simulink model "jessilll"  (R2021a)
settings: Solver=VariableStepAuto  StartTime=0.0  StopTime=500  RelTol=1e-3
settings Model: Creator=USER  LastModifiedBy=User

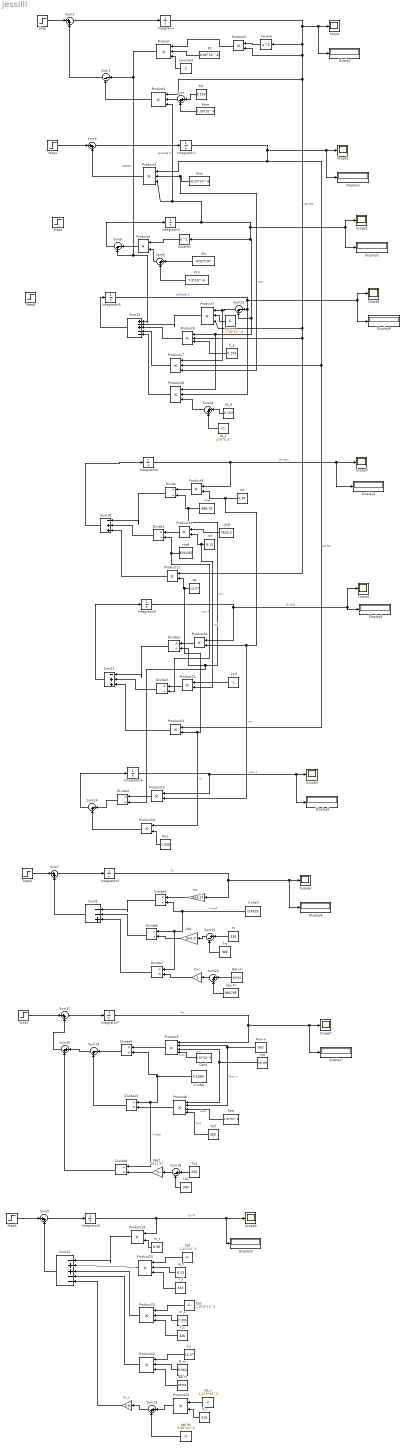
== system jessilll ==
  Constant : Constant  Value=2
  Cp_v : Constant  Value=2.373*10^3
  Cpc : Constant  Value=1.814*10^3
  Cpf : Constant  Value=1.22*10^3
  Cpv Tr : Constant  Value=984795
  Cpw : Constant  Value=1.87*10^3
  Cpw1 : Constant  Value=1.87*10^3
  Del Hv : Constant  Value=69781
  Display{,1..9} (10 alike) : Display
  Divide{,1..5,9} (7 alike) : Product  Inputs=*/
  Divide{6..8,10} (4 alike) : Product  Inputs=/*
  Integrator{,1..2,6..9} (7 alike) : Integrator
  Integrator3 : Integrator  InitialCondition=415
  Integrator4 : Integrator  InitialCondition=7632.2
  Integrator5 : Integrator  InitialCondition=587.47
  K_p : Constant  Value=0.193
  Kp : Constant  Value=0.193
  Kt_c : Constant  Value=47075.07
  Kt_d : Constant  Value=0.193
  Ktc : Constant  Value=47075.07
  Ktd : Constant  Value=7.3*10^-6
  Kti : Constant  Value=8.86*10^-20
  Ktrm : Constant  Value=7.39*10^-6
  Ktrm_1 : Constant  Value=7.39*10^-6
  Ktrs : Constant  Value=-8.25*10^-6
  Product{,1,3,7..8,17..18,20..22} (10 alike) : Product  Inputs=3
  Product{2,4,9..16,19,23} (12 alike) : Product
  Product5 : Product  Inputs=4
  Product6 : Product  Inputs=4
  R_m : Constant  Value=8.964
  Row w : Constant  Value=997
  Ru1 : Constant  Value=1.008
  Scope{,1..9} (10 alike) : Scope
  Square : Math  Operator=square  SaturateOnIntegerOverflow=on
  Square1 : Math  Operator=square  SaturateOnIntegerOverflow=on
  Step : Step  Time=0  Before=0.001  After=0.25  SampleTime=0
  Step1 : Step  Time=0  Before=0.001  After=0.01  SampleTime=0
  Step{2..4,8} (4 alike) : Step  SampleTime=0
  Step7 : Step  After=326  SampleTime=0
  Sum{,2..3,5,7,9,13,16..17,20,24} (11 alike) : Sum  Inputs=|++
  Sum1 : Sum  Inputs=|--
  Sum10 : Sum  Inputs=|-++
  Sum11 : Sum  Inputs=|-++
  Sum12 : Sum  Inputs=|-++--
  Sum{6,14,19,22} (4 alike) : Sum  Inputs=|-+
  Sum15 : Sum  Inputs=|+-
  Sum18 : Sum  Inputs=|+-
  Sum23 : Sum  Inputs=|+-+--
  Sum8 : Sum  Inputs=|--+
  T_c : Constant  Value=326
  T_f : Constant  Value=333
  T_r : Constant  Value=415
  Tc : Constant  Value=326
  Tc1 : Constant  Value=326
  Tw : Constant  Value=300
  Tw1 : Constant  Value=300
  Twf : Constant  Value=300
  UAc : Gain  Gain=3842.37
  UAc1 : Gain  Gain=3842.37
  V shell : Constant  Value=0.4919
  V tube : Constant  Value=0.1094
  VR : Constant  Value=14.07
  V_r : Constant  Value=14.07
  "[M]f" : Constant  Value=7632.2
  "[S]f" : Constant
  del H : Constant  Value=69781
  del Hv : Constant  Value=6.99*10^4
  m_c : Constant  Value=0.305
  m_f : Constant  Value=6.13
  m_t : Constant  Value=6.39
  m_v : Gain  Gain=3.96
  mc : Gain  Gain=553.27
  mf : Constant  Value=6.13
  mt : Constant  Value=6.39
  mv : Gain
  mw : Constant  Value=59.09
  row : Constant  Value=986.76
  rowf : Constant  Value=858.085
  wires:
  Integrator/1 -> Display/1, Scope/1, Product7/3, Product8/2, Product11/1, Product1/1, Product2/2, Square/1  "[M] RM"
  Kti/1 -> Product/2
  Constant/1 -> Product/3
  Kp/1 -> Sum/1
  Ktrm/1 -> Sum/2
  Sum/1 -> Product1/2
  Product/1 -> Sum6/2, Sum23/1, Sum1/1  "2Kti[M]"
  Product1/1 -> Sum1/2
  Square/1 -> Product2/1
  Product2/1 -> Product/1
  Sum1/1 -> Sum2/2
  Step/1 -> Sum2/1
  Sum2/1 -> Integrator/1
  Step1/1 -> Sum3/1
  Sum3/1 -> Integrator1/1
  Integrator1/1 -> Product3/1, Product17/2, Product13/1, Display1/1, Scope1/1  "[S] RS"
  Ktrs/1 -> Product17/3, Product3/2  "Ktrs"
  Product3/1 -> Sum3/2
  Sum6/1 -> Integrator2/1
  Integrator2/1 -> Product1/3, Product3/3, Scope2/1, Display2/1, Square1/1, Product18/1, Product8/1, Sum22/2  "Lambda 0"
  Ktc/1 -> Sum5/1
  Ktd/1 -> Sum5/2
  Square1/1 -> Product4/1
  Sum5/1 -> Product4/2
  Product4/1 -> Sum6/1
  Sum10/1 -> Integrator4/1
  Product9/1 -> Divide/1
  mf/1 -> Product12/2, Product10/2  "mf"
  Product10/1 -> Divide1/1
  rowf/1 -> Divide3/2, Divide1/2  "row f"
  "[M]f"/1 -> Product10/1
  VR/1 -> Product16/1, Product13/2, Product11/2  "Vr"
  Divide/1 -> Sum10/1
  Divide1/1 -> Sum10/2
  Product11/1 -> Sum10/3
  Divide2/1 -> Sum11/1
  Sum11/1 -> Integrator5/1
  row/1 -> Divide/2, Divide4/2, Divide2/2  "row"
  Product13/1 -> Sum11/3
  Divide3/1 -> Sum11/2
  mt/1 -> Product9/2, Product15/2, Product14/2  "mt"
  Product14/1 -> Divide2/1
  Product12/1 -> Divide3/1
  Sum14/1 -> Integrator6/1
  "[S]f"/1 -> Product12/1
  Product15/1 -> Divide4/1
  Divide4/1 -> Sum14/1
  Product16/1 -> Sum14/2
  Ru1/1 -> Product16/2
  Step3/1 -> Sum7/1
  Sum7/1 -> Integrator3/1
  mc/1 -> Divide5/1
  Integrator3/1 -> Display6/1, Scope6/1, mc/1  "Tc"
  V shell/1 -> Divide6/1, Divide7/1, Divide5/2  "V shell"
  Divide5/1 -> Sum8/1
  Tw/1 -> Sum15/2
  Tc/1 -> Sum15/1
  UAc/1 -> Divide6/2
  Sum15/1 -> UAc/1
  Divide6/1 -> Sum8/2
  Del Hv/1 -> Sum16/1
  Cpv Tr/1 -> Sum16/2
  mv/1 -> Divide7/2
  Sum16/1 -> mv/1
  Sum8/1 -> Sum7/2
  Step7/1 -> Sum17/1
  Sum17/1 -> Integrator7/1
  Divide7/1 -> Sum8/3
  Tc1/1 -> Sum18/1
  Tw1/1 -> Sum18/2
  UAc1/1 -> Divide8/2
  Sum18/1 -> UAc1/1
  Integrator4/1 -> Product9/1, Scope3/1, Display3/1  "[M dot]"
  Integrator5/1 -> Product14/1, Scope4/1, Display4/1  "[S dot]"
  Integrator6/1 -> Display5/1, Scope5/1, Product15/1  "meu 1"
  Integrator7/1 -> Display7/1, Scope7/1, Product5/1  "Tw"
  Row w/1 -> Product6/2, Product5/2  "Row w"
  mw/1 -> Product6/1, Product5/3  "mw"
  Product5/1 -> Divide9/1
  V tube/1 -> Divide9/2, Divide8/1, Divide10/1  "V tube"
  Divide9/1 -> Sum19/1
  Cpw/1 -> Product6/3  "Cpw"
  Twf/1 -> Product6/4  "Twf"
  Product6/1 -> Divide10/2
  Divide10/1 -> Sum19/2
  Sum20/1 -> Sum17/2
  Sum19/1 -> Sum20/1
  Divide8/1 -> Sum20/2
  Sum23/1 -> Integrator8/1
  Integrator8/1 -> Scope8/1, Display8/1, Product18/2, Sum22/1  "Lambda 1"
  Sum22/1 -> Product17/1, Product7/1
  Ktrm_1/1 -> Product7/2
  Product7/1 -> Sum23/2
  K_p/1 -> Product8/3
  Product8/1 -> Sum23/3
  Product17/1 -> Sum23/4
  Product18/1 -> Sum23/5
  Kt_c/1 -> Sum24/2
  Kt_d/1 -> Sum24/1
  Sum24/1 -> Product18/3
  Step4/1 -> Sum9/1
  Sum9/1 -> Integrator9/1
  Integrator9/1 -> Product19/1, Display9/1, Scope9/1  "Cp Tr"
  m_t/1 -> Product19/2
  Product19/1 -> Sum12/1
  T_f/1 -> Product20/3
  m_f/1 -> Product20/2
  Cpf/1 -> Product20/1
  Product20/1 -> Sum12/2
  Cpc/1 -> Product21/1
  m_c/1 -> Product21/2
  T_c/1 -> Product21/3
  Product21/1 -> Sum12/3
  V_r/1 -> Product22/1
  R_m/1 -> Product22/2
  del H/1 -> Product22/3
  Product22/1 -> Sum12/4
  Cp_v/1 -> Product23/1
  T_r/1 -> Product23/2
  Product23/1 -> Sum13/1
  del Hv/1 -> Sum13/2
  Sum13/1 -> m_v/1
  m_v/1 -> Sum12/5
  Sum12/1 -> Sum9/2
  Cpw1/1 -> Product5/4  "Cpw"
